simulink model "Simulink_6"  (R2016b)
settings: Solver=VariableStepAuto  StartTime=0.0  StopTime=70  RelTol=1e-3
values from neighbouring files (symbols this model uses):
  C_lon = [1 0 0 0 ... (first row only)    [ejercicio07_longitudinal_C.m]
  D_lon = zeros(2)    [ejercicio07_longitudinal_C.m]
  delta_e_dot_lim = [-90 90]    [ejercicio07_lateral_C.m]    (also in ejercicio07_longitudinal_C.m)
  delta_e_lim = [-25 25]    [ejercicio07_lateral_C.m]    (also in ejercicio07_longitudinal_C.m)
  delta_th_dot_lim = [-0.24 0.24]*100    [ejercicio07_lateral_C.m]    (also in ejercicio07_longitudinal_C.m)
  delta_th_lim = [-0.2 0.8]*100    [ejercicio07_lateral_C.m]    (also in ejercicio07_longitudinal_C.m)
  dt = 0.001    [ejercicio07_lateral_C.m]    (also in ejercicio07_longitudinal_C.m)
  F_lon = A_lon*Tm + I    [ejercicio07_longitudinal_C.m]
  G_lon = B_lon*Tm    [ejercicio07_longitudinal_C.m]
  Kc = Kc_a(:,1:4)    [ejercicio07_lateral_C.m]    (also in ejercicio07_longitudinal_C.m)
  Ki = -Kc_a(:,5:6)    [ejercicio07_lateral_C.m]    (also in ejercicio07_longitudinal_C.m)
  Ko_d = dlqe(F_lat,G_lat,C_lat,V1,V2)    [ejercicio07_lateral_C.m]    (also in ejercicio07_longitudinal_C.m = dlqe(F_lon,G_lon,C_lon,V1,V2))
  PreC = [Cyr*(I-Fyr)^(-1)*G_lat+D_lat]^(-1)    [ejercicio07_lateral_C.m]    (also in ejercicio07_longitudinal_C.m = [Cyr*(I-Fyr)^(-1)*G_lon+D_lon]^(-1))
  tau_e = 1/20    (= 0.05)    [ejercicio07_longitudinal_C.m]
  tau_th = 0.5    [ejercicio07_longitudinal_C.m]
  Tm = 0.003    [ejercicio07_lateral_C.m]    (also in ejercicio07_longitudinal_C.m)
undefined symbols (not defined in the file or in its folder): DiscIntNeverNeededParam, Ko
undefined symbols (not defined in the file): sys_lon
(part 3 of 3)

== system Simulink_6/Ejercicio 6/EJERCICIO 6 DISCRETO/Comparativa ejercicio 6/Comparativa modal/CONTROL LONGITUDINAL CONTINUA/ACTUADORES/ELEVADOR ==
  u_e : Inport
  Fpdot1 : Saturate  UpperLimit=delta_e_dot_lim(2)  LowerLimit=delta_e_dot_lim(1)
  Integrator4 : Integrator  LimitOutput=on  UpperSaturationLimit=delta_e_lim(2)  LowerSaturationLimit=delta_e_lim(1)
  KT/taup3 : Gain  Gain=1/tau_e
  Km9 : Gain  Gain=1/tau_e
  Sum10 : Sum  Inputs=|+-
  delta_e : Outport
  wires:
  Km9/1 -> Sum10/2
  Integrator4/1 -> Km9/1, delta_e/1  "delta_e"
  Sum10/1 -> Fpdot1/1  "delta_e_dot"
  KT/taup3/1 -> Sum10/1
  Fpdot1/1 -> Integrator4/1
  u_e/1 -> KT/taup3/1

== system Simulink_6/Ejercicio 6/EJERCICIO 6 DISCRETO/Comparativa ejercicio 6/Comparativa modal/CONTROL LONGITUDINAL CONTINUA/ACTUADORES/THROTTLE ==
  u_th : Inport
  Fpdot1 : Saturate  UpperLimit=delta_th_dot_lim(2)  LowerLimit=delta_th_dot_lim(1)
  Integrator4 : Integrator  LimitOutput=on  UpperSaturationLimit=delta_th_lim(2)  LowerSaturationLimit=delta_th_lim(1)
  KT/taup3 : Gain  Gain=1/tau_th
  Km9 : Gain  Gain=1/tau_th
  Sum10 : Sum  Inputs=|+-
  delta_th : Outport
  wires:
  Km9/1 -> Sum10/2
  Integrator4/1 -> Km9/1, delta_th/1  "delta_th"
  Sum10/1 -> Fpdot1/1  "delta_th_dot"
  KT/taup3/1 -> Sum10/1
  Fpdot1/1 -> Integrator4/1
  u_th/1 -> KT/taup3/1

== system Simulink_6/Ejercicio 6/EJERCICIO 6 DISCRETO/Comparativa ejercicio 6/Comparativa modal/CONTROL LONGITUDINAL DISCRETO/ACTUADORES/ELEVADOR ==
  u_e : Inport
  Fpdot1 : Saturate  UpperLimit=delta_e_dot_lim(2)  LowerLimit=delta_e_dot_lim(1)
  Integrator4 : Integrator  LimitOutput=on  UpperSaturationLimit=delta_e_lim(2)  LowerSaturationLimit=delta_e_lim(1)
  KT/taup3 : Gain  Gain=1/tau_e
  Km9 : Gain  Gain=1/tau_e
  Sum10 : Sum  Inputs=|+-
  delta_e : Outport
  wires:
  Km9/1 -> Sum10/2
  Integrator4/1 -> Km9/1, delta_e/1  "delta_e"
  Sum10/1 -> Fpdot1/1  "delta_e_dot"
  KT/taup3/1 -> Sum10/1
  Fpdot1/1 -> Integrator4/1
  u_e/1 -> KT/taup3/1

== system Simulink_6/Ejercicio 6/EJERCICIO 6 DISCRETO/Comparativa ejercicio 6/Comparativa modal/CONTROL LONGITUDINAL DISCRETO/ACTUADORES/THROTTLE ==
  u_th : Inport
  Fpdot1 : Saturate  UpperLimit=delta_th_dot_lim(2)  LowerLimit=delta_th_dot_lim(1)
  Integrator4 : Integrator  LimitOutput=on  UpperSaturationLimit=delta_th_lim(2)  LowerSaturationLimit=delta_th_lim(1)
  KT/taup3 : Gain  Gain=1/tau_th
  Km9 : Gain  Gain=1/tau_th
  Sum10 : Sum  Inputs=|+-
  delta_th : Outport
  wires:
  Km9/1 -> Sum10/2
  Integrator4/1 -> Km9/1, delta_th/1  "delta_th"
  Sum10/1 -> Fpdot1/1  "delta_th_dot"
  KT/taup3/1 -> Sum10/1
  Fpdot1/1 -> Integrator4/1
  u_th/1 -> KT/taup3/1

== system Simulink_6/Ejercicio 6/EJERCICIO 6 DISCRETO/Comparativa ejercicio 7/Comparativa Integral/CONTROL LONGITUDINAL DISCRETO ACCION INTEGRAL/ACTUADORES/ELEVADOR ==
  u_e : Inport
  Fpdot1 : Saturate  UpperLimit=delta_e_dot_lim(2)  LowerLimit=delta_e_dot_lim(1)
  Integrator4 : Integrator  LimitOutput=on  UpperSaturationLimit=delta_e_lim(2)  LowerSaturationLimit=delta_e_lim(1)
  KT/taup3 : Gain  Gain=1/tau_e
  Km9 : Gain  Gain=1/tau_e
  Sum10 : Sum  Inputs=|+-
  delta_e : Outport
  wires:
  Km9/1 -> Sum10/2
  Integrator4/1 -> Km9/1, delta_e/1  "delta_e"
  Sum10/1 -> Fpdot1/1  "delta_e_dot"
  KT/taup3/1 -> Sum10/1
  Fpdot1/1 -> Integrator4/1
  u_e/1 -> KT/taup3/1

== system Simulink_6/Ejercicio 6/EJERCICIO 6 DISCRETO/Comparativa ejercicio 7/Comparativa Integral/CONTROL LONGITUDINAL DISCRETO ACCION INTEGRAL/ACTUADORES/THROTTLE ==
  u_th : Inport
  Fpdot1 : Saturate  UpperLimit=delta_th_dot_lim(2)  LowerLimit=delta_th_dot_lim(1)
  Integrator4 : Integrator  LimitOutput=on  UpperSaturationLimit=delta_th_lim(2)  LowerSaturationLimit=delta_th_lim(1)
  KT/taup3 : Gain  Gain=1/tau_th
  Km9 : Gain  Gain=1/tau_th
  Sum10 : Sum  Inputs=|+-
  delta_th : Outport
  wires:
  Km9/1 -> Sum10/2
  Integrator4/1 -> Km9/1, delta_th/1  "delta_th"
  Sum10/1 -> Fpdot1/1  "delta_th_dot"
  KT/taup3/1 -> Sum10/1
  Fpdot1/1 -> Integrator4/1
  u_th/1 -> KT/taup3/1

== system Simulink_6/Ejercicio 6/EJERCICIO 6 DISCRETO/Comparativa ejercicio 7/Comparativa Integral/CONTROL LONGITUDINAL DISCRETO ACCION INTEGRAL1/ACTUADORES/ELEVADOR ==
  u_e : Inport
  Fpdot1 : Saturate  UpperLimit=delta_e_dot_lim(2)  LowerLimit=delta_e_dot_lim(1)
  Integrator4 : Integrator  LimitOutput=on  UpperSaturationLimit=delta_e_lim(2)  LowerSaturationLimit=delta_e_lim(1)
  KT/taup3 : Gain  Gain=1/tau_e
  Km9 : Gain  Gain=1/tau_e
  Sum10 : Sum  Inputs=|+-
  delta_e : Outport
  wires:
  Km9/1 -> Sum10/2
  Integrator4/1 -> Km9/1, delta_e/1  "delta_e"
  Sum10/1 -> Fpdot1/1  "delta_e_dot"
  KT/taup3/1 -> Sum10/1
  Fpdot1/1 -> Integrator4/1
  u_e/1 -> KT/taup3/1

== system Simulink_6/Ejercicio 6/EJERCICIO 6 DISCRETO/Comparativa ejercicio 7/Comparativa Integral/CONTROL LONGITUDINAL DISCRETO ACCION INTEGRAL1/ACTUADORES/THROTTLE ==
  u_th : Inport
  Fpdot1 : Saturate  UpperLimit=delta_th_dot_lim(2)  LowerLimit=delta_th_dot_lim(1)
  Integrator4 : Integrator  LimitOutput=on  UpperSaturationLimit=delta_th_lim(2)  LowerSaturationLimit=delta_th_lim(1)
  KT/taup3 : Gain  Gain=1/tau_th
  Km9 : Gain  Gain=1/tau_th
  Sum10 : Sum  Inputs=|+-
  delta_th : Outport
  wires:
  Km9/1 -> Sum10/2
  Integrator4/1 -> Km9/1, delta_th/1  "delta_th"
  Sum10/1 -> Fpdot1/1  "delta_th_dot"
  KT/taup3/1 -> Sum10/1
  Fpdot1/1 -> Integrator4/1
  u_th/1 -> KT/taup3/1

== system Simulink_6/Ejercicio 6/EJERCICIO 6 DISCRETO/Comparativa ejercicio 7/Comparativa modal/CONTROL LONGITUDINAL DISCRETO EJERCICIO 6/ACTUADORES/ELEVADOR ==
  u_e : Inport
  Fpdot1 : Saturate  UpperLimit=delta_e_dot_lim(2)  LowerLimit=delta_e_dot_lim(1)
  Integrator4 : Integrator  LimitOutput=on  UpperSaturationLimit=delta_e_lim(2)  LowerSaturationLimit=delta_e_lim(1)
  KT/taup3 : Gain  Gain=1/tau_e
  Km9 : Gain  Gain=1/tau_e
  Sum10 : Sum  Inputs=|+-
  delta_e : Outport
  wires:
  Km9/1 -> Sum10/2
  Integrator4/1 -> Km9/1, delta_e/1  "delta_e"
  Sum10/1 -> Fpdot1/1  "delta_e_dot"
  KT/taup3/1 -> Sum10/1
  Fpdot1/1 -> Integrator4/1
  u_e/1 -> KT/taup3/1

== system Simulink_6/Ejercicio 6/EJERCICIO 6 DISCRETO/Comparativa ejercicio 7/Comparativa modal/CONTROL LONGITUDINAL DISCRETO EJERCICIO 6/ACTUADORES/THROTTLE ==
  u_th : Inport
  Fpdot1 : Saturate  UpperLimit=delta_th_dot_lim(2)  LowerLimit=delta_th_dot_lim(1)
  Integrator4 : Integrator  LimitOutput=on  UpperSaturationLimit=delta_th_lim(2)  LowerSaturationLimit=delta_th_lim(1)
  KT/taup3 : Gain  Gain=1/tau_th
  Km9 : Gain  Gain=1/tau_th
  Sum10 : Sum  Inputs=|+-
  delta_th : Outport
  wires:
  Km9/1 -> Sum10/2
  Integrator4/1 -> Km9/1, delta_th/1  "delta_th"
  Sum10/1 -> Fpdot1/1  "delta_th_dot"
  KT/taup3/1 -> Sum10/1
  Fpdot1/1 -> Integrator4/1
  u_th/1 -> KT/taup3/1

== system Simulink_6/Ejercicio 6/EJERCICIO 6 DISCRETO/Comparativa ejercicio 7/Comparativa modal/CONTROL LONGITUDINAL DISCRETO EJERCICIO 7/ACTUADORES/ELEVADOR ==
  u_e : Inport
  Fpdot1 : Saturate  UpperLimit=delta_e_dot_lim(2)  LowerLimit=delta_e_dot_lim(1)
  Integrator4 : Integrator  LimitOutput=on  UpperSaturationLimit=delta_e_lim(2)  LowerSaturationLimit=delta_e_lim(1)
  KT/taup3 : Gain  Gain=1/tau_e
  Km9 : Gain  Gain=1/tau_e
  Sum10 : Sum  Inputs=|+-
  delta_e : Outport
  wires:
  Km9/1 -> Sum10/2
  Integrator4/1 -> Km9/1, delta_e/1  "delta_e"
  Sum10/1 -> Fpdot1/1  "delta_e_dot"
  KT/taup3/1 -> Sum10/1
  Fpdot1/1 -> Integrator4/1
  u_e/1 -> KT/taup3/1

== system Simulink_6/Ejercicio 6/EJERCICIO 6 DISCRETO/Comparativa ejercicio 7/Comparativa modal/CONTROL LONGITUDINAL DISCRETO EJERCICIO 7/ACTUADORES/THROTTLE ==
  u_th : Inport
  Fpdot1 : Saturate  UpperLimit=delta_th_dot_lim(2)  LowerLimit=delta_th_dot_lim(1)
  Integrator4 : Integrator  LimitOutput=on  UpperSaturationLimit=delta_th_lim(2)  LowerSaturationLimit=delta_th_lim(1)
  KT/taup3 : Gain  Gain=1/tau_th
  Km9 : Gain  Gain=1/tau_th
  Sum10 : Sum  Inputs=|+-
  delta_th : Outport
  wires:
  Km9/1 -> Sum10/2
  Integrator4/1 -> Km9/1, delta_th/1  "delta_th"
  Sum10/1 -> Fpdot1/1  "delta_th_dot"
  KT/taup3/1 -> Sum10/1
  Fpdot1/1 -> Integrator4/1
  u_th/1 -> KT/taup3/1

== matlab function Simulink_6/Ejercicio 6/EJERCICIO 6 DISCRETO/CONTROL LONGITUDINALDISCRETO FBW/Computador digital/Algoritmo de control ==
  settings: updateMethod=DISCRETE  sampleTime=Tm
  data: Tm input; F input; G input; C input; D input; CO output; Ki input; Kc input; K_od input; sp input; y input; mv input size=2; SPF output
function [CO, SPF] = fcn(Tm, F, G, C, D, Ki, Kc, K_od, sp, y, mv)

    persistent vT_sp_a RSR FSR tau_f int_error error_a xe

    if isempty(vT_sp_a)
        vT_sp_a = sp(1);
        RSR = 3;
        FSR = -3;
        tau_f = 1;
        int_error = [0 0]';
        error_a = [0 0]';
        xe=[0 0 0 0]';
    end    

    vT_sp = sp(1);
    rate = (vT_sp - vT_sp_a)/Tm;

    if rate > RSR
        vT_spf = RSR*Tm+vT_sp_a;
    elseif rate < FSR
        vT_spf = FSR*Tm+vT_sp_a;
    else
        vT_spf = vT_sp;
    end

    vT_spf_a = (1-Tm/tau_f)*vT_spf+(Tm/tau_f)*vT_spf;
    vT_sp_a = vT_spf;

    spf = [vT_spf sp(2)]';
    error = spf - y;
    
    int_error = int_error + (error + error_a)*Tm/2; 
    error_a = error;

    ye = C*xe + D*mv;
    xe = F*xe + G*mv+K_od*(y-ye);    
  
    u = Ki*int_error-Kc*xe;

    CO = u;
    SPF = spf;

== matlab function Simulink_6/Ejercicio 6/EJERCICIO 6 DISCRETO/CONTROL LONGITUDINALDISCRETO FBW (ACCION INTEGRAL)/Computador digital/Algoritmo de control ==
  settings: updateMethod=DISCRETE  sampleTime=Tm
  data: Tm input; F input; G input; C input; D input; CO output; Ki input; Kc input; K_od input; sp input; y input; mv input size=2; SPF output
function [CO, SPF] = fcn(Tm, F, G, C, D, Ki, Kc, K_od, sp, y, mv)

    persistent vT_sp_a RSR FSR tau_f int_error error_a xe

    if isempty(vT_sp_a)
        vT_sp_a = sp(1);
        RSR = 3;
        FSR = -3;
        tau_f = 1;
        int_error = [0 0]';
        error_a = [0 0]';
        xe=[0 0 0 0]';
    end    

    vT_sp = sp(1);
    rate = (vT_sp - vT_sp_a)/Tm;

    if rate > RSR
        vT_spf = RSR*Tm+vT_sp_a;
    elseif rate < FSR
        vT_spf = FSR*Tm+vT_sp_a;
    else
        vT_spf = vT_sp;
    end

    vT_spf_a = (1-Tm/tau_f)*vT_spf+(Tm/tau_f)*vT_spf;
    vT_sp_a = vT_spf;

    spf = [vT_spf sp(2)]';
    error = spf - y;
    
    int_error = int_error + (error + error_a)*Tm/2; 
    error_a = error;

    ye = C*xe + D*mv;
    xe = F*xe + G*mv+K_od*(y-ye);    
  
    u = Ki*int_error-Kc*xe;

    CO = u;
    SPF = spf;
